simulink model "converting_binary"  (R2019b)
settings: Solver=VariableStepAuto  StartTime=0.0  StopTime=10  RelTol=1e-3
undefined symbols (not defined in the file or in its folder): serial
libraries: instrumentlib x3
settings Model: Creator=hirolab  LastModifiedBy=hirolab

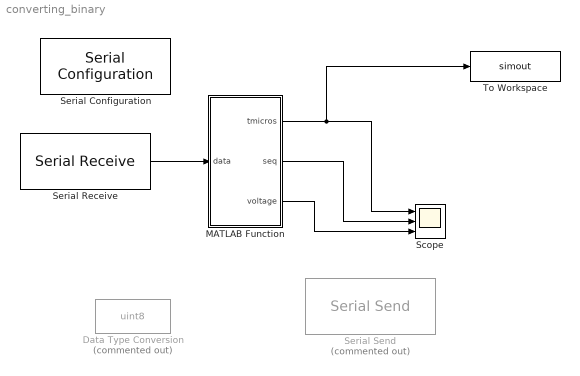
== system converting_binary ==
  Data Type Conversion : DataTypeConversion  Commented=on  OutDataTypeStr=uint8
  MATLAB Function : MATLAB Function  TreatAsAtomicUnit=on
  Scope : Scope  NumInputPorts=3
  Serial Configuration : instrumentlib/Serial Configuration  Priority=-200000  ComPortMenu=COM3  ComPort=COM3  ObjConstructor=serial('COM3');  BaudRate=9600  DataBits=8  Parity=none  StopBits=1  FlowControl=none  Timeout=10  ByteOrder=LittleEndian
  Serial Receive : instrumentlib/Serial Receive  ComPortMenu=COM3  ComPort=COM3  ObjConstructor=serial('COM3');  Header=sop  Terminator=<none>  DataSize="[12  100]"  DataType=uint8  EnableBlockingMode=on  ActionDataUnavailable=Output last received value  CustomValue=0  SampleTime=.1
  Serial Send : instrumentlib/Serial Send  Commented=on  ComPortMenu=<Please select a port...>  ComPort=<Please select a port...>  Terminator=<none>  EnableBlockingMode=on
  To Workspace : ToWorkspace  VariableName=simout  SaveFormat=Timeseries  SampleTime=-1
  wires:
  Serial Receive/1 -> MATLAB Function/1(data)
  MATLAB Function/3(voltage) -> Scope/3
  MATLAB Function/2(seq) -> Scope/2
  MATLAB Function/1(tmicros) -> Scope/1, To Workspace/1

== matlab function converting_binary/MATLAB Function ==
  data: data input uint8; tmicros output; seq output; voltage output
function [tmicros, seq, voltage] = fcn(data)
% REMINDER edit_data > change input data to unit8

block_size = 100;
tmicros = zeros(block_size, 1);
seq = zeros(block_size,1);
voltage = zeros(block_size, 1);

for i = 1 : block_size 
tmicros(i,:) = typecast(data(1:4,i), 'uint32')*1*10^-6;
seq(i,:) = typecast(data(5:8,i), 'int32');
voltage(i,:) = typecast(data(9:12,i ), 'single');

end
